simulink model "Sensorverwerking_case1"  (R2018b)
settings: Solver=VariableStepAuto  StartTime=0.0  StopTime=10.0  RelTol=1e-3
undefined symbols (not defined in the file or in its folder): n, sigbuilder_block, Tsc
libraries: dspswit3 x10, simulink x7, powerlib_meascontrol x4, dspsigops x4, peGeneralControl x1
settings Model: Creator=Roberto  LastModifiedBy=Roberto

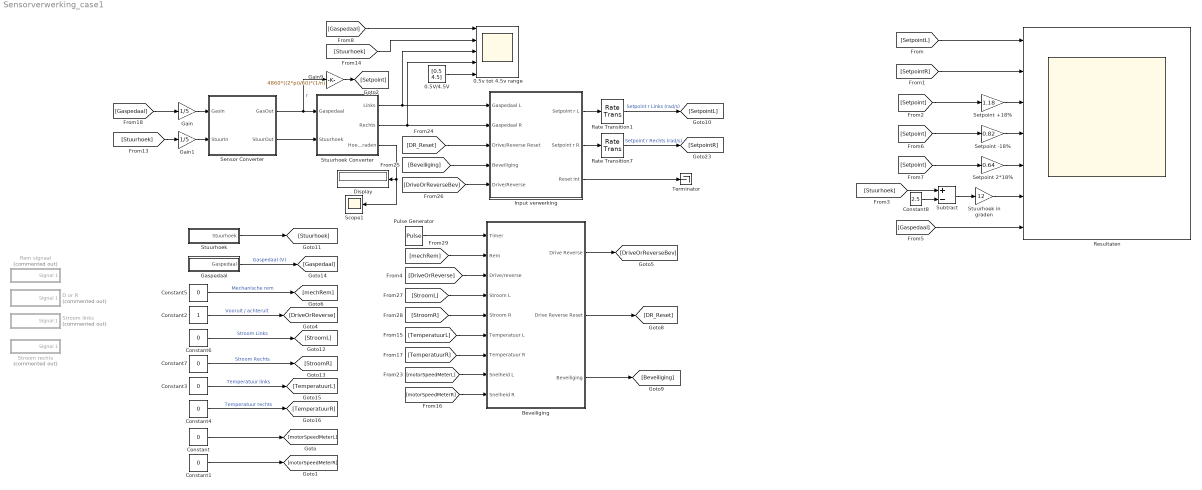
== system Sensorverwerking_case1 ==
  0.5V/4.5V : Constant  Value=[0.5 4.5]
  0.5v tot 4.5v range : Scope  NumInputPorts=5
  Beveiliging : Subsystem
  Constant{,1,3..7} (7 alike) : Constant  Value=0
  Constant2 : Constant
  Constant8 : Constant  Value=2.5
  D or R : Subsystem  Tag=STV Subsys  Commented=on  LoadFcn=sigbuilder_block('load');  StartFcn=sigbuilder_block('start');  StopFcn=sigbuilder_block('stop');  ClipboardFcn=sigbuilder_block('clipboard');  mask(Sigbuilder block){tuvar=[0:10]}
      mask help: Simulink:masks:SigbuilderBlock_MD
      mask init:
      | if ~strcmp(get_param(bdroot(gcbh),'SimulationStatus'),'stopped') tuvar = sigbuilder_block('maskInit'); end
      settings: CopyFcn=sigbuilder_block('copy');  DeleteFcn=sigbuilder_block('delete');  ModelCloseFcn=sigbuilder_block('modelClose');  PreSaveFcn=sigbuilder_block('preSave');  PauseFcn=sigbuilder_block('pause');  ContinueFcn=sigbuilder_block('continue');  NameChangeFcn=sigbuilder_block('namechange');  OpenFcn=sigbuilder_block('open',[437.6 153 550.4 359.25 ]);  CloseFcn=sigbuilder_block('close');
      mask Display: plot(0, 0, 100, 100,[2, 2, 32, 32, 2], [68, 8, 8, 68, 68],[32, 2], [38, 38], [32, 19, 2],[53, 60, 44], [32, 17, 17, 2],[16, 16, 31, 31]);txt = getActiveGroup(gcbh);text(2, 100, txt,'verticalAlignment', 'top');
  Display : Display
  Gain : Gain  Gain=1/5
  Gain1 : Gain  Gain=1/5
  Gain9 : Gain  Gain=4860*((2*pi)/60)*(1/n)
  Gaspedaal : Subsystem  Tag=STV Subsys  LoadFcn=sigbuilder_block('load');  StartFcn=sigbuilder_block('start');  StopFcn=sigbuilder_block('stop');  ClipboardFcn=sigbuilder_block('clipboard');  mask(Sigbuilder block){tuvar=[0:10]}
      mask help: Simulink:masks:SigbuilderBlock_MD
      mask init:
      | if ~strcmp(get_param(bdroot(gcbh),'SimulationStatus'),'stopped') tuvar = sigbuilder_block('maskInit'); end
      settings: CopyFcn=sigbuilder_block('copy');  DeleteFcn=sigbuilder_block('delete');  ModelCloseFcn=sigbuilder_block('modelClose');  PreSaveFcn=sigbuilder_block('preSave');  PauseFcn=sigbuilder_block('pause');  ContinueFcn=sigbuilder_block('continue');  NameChangeFcn=sigbuilder_block('namechange');  OpenFcn=sigbuilder_block('open',[468 234 550.5 278.25 ]);  CloseFcn=sigbuilder_block('close');
      mask Display: plot(0, 0, 100, 100,[2, 2, 32, 32, 2], [68, 8, 8, 68, 68],[32, 2], [38, 38], [32, 19, 2],[53, 60, 44], [32, 17, 17, 2],[16, 16, 31, 31]);txt = getActiveGroup(gcbh);text(2, 100, txt,'verticalAlignment', 'top');
  Input verwerking : Subsystem
  Pulse Generator : DiscretePulseGenerator  SampleTime=1/2000
  Rate Transition1 : RateTransition  OutPortSampleTime=Tsc
  Rate Transition7 : RateTransition  OutPortSampleTime=Tsc
  Rem signaal : Subsystem  Tag=STV Subsys  Commented=on  LoadFcn=sigbuilder_block('load');  StartFcn=sigbuilder_block('start');  StopFcn=sigbuilder_block('stop');  ClipboardFcn=sigbuilder_block('clipboard');  mask(Sigbuilder block){tuvar=[0:10]}
      mask help: Simulink:masks:SigbuilderBlock_MD
      mask init:
      | if ~strcmp(get_param(bdroot(gcbh),'SimulationStatus'),'stopped') tuvar = sigbuilder_block('maskInit'); end
      settings: CopyFcn=sigbuilder_block('copy');  DeleteFcn=sigbuilder_block('delete');  ModelCloseFcn=sigbuilder_block('modelClose');  PreSaveFcn=sigbuilder_block('preSave');  PauseFcn=sigbuilder_block('pause');  ContinueFcn=sigbuilder_block('continue');  NameChangeFcn=sigbuilder_block('namechange');  OpenFcn=sigbuilder_block('open',[437.6 153 550.4 359.25 ]);  CloseFcn=sigbuilder_block('close');
      mask Display: plot(0, 0, 100, 100,[2, 2, 32, 32, 2], [68, 8, 8, 68, 68],[32, 2], [38, 38], [32, 19, 2],[53, 60, 44], [32, 17, 17, 2],[16, 16, 31, 31]);txt = getActiveGroup(gcbh);text(2, 100, txt,'verticalAlignment', 'top');
  Resultaten : Scope  NumInputPorts=7
  Scope1 : Scope
  Sensor Converter : Subsystem
  Setpoint +18% : Gain  Gain=1.18
  Setpoint -18% : Gain  Gain=0.82
  Setpoint 2*18% : Gain  Gain=0.64
  Stroom links : Subsystem  Tag=STV Subsys  Commented=on  LoadFcn=sigbuilder_block('load');  StartFcn=sigbuilder_block('start');  StopFcn=sigbuilder_block('stop');  ClipboardFcn=sigbuilder_block('clipboard');  mask(Sigbuilder block){tuvar=[0:10]}
      mask help: Simulink:masks:SigbuilderBlock_MD
      mask init:
      | if ~strcmp(get_param(bdroot(gcbh),'SimulationStatus'),'stopped') tuvar = sigbuilder_block('maskInit'); end
      settings: CopyFcn=sigbuilder_block('copy');  DeleteFcn=sigbuilder_block('delete');  ModelCloseFcn=sigbuilder_block('modelClose');  PreSaveFcn=sigbuilder_block('preSave');  PauseFcn=sigbuilder_block('pause');  ContinueFcn=sigbuilder_block('continue');  NameChangeFcn=sigbuilder_block('namechange');  OpenFcn=sigbuilder_block('open',[437.6 153 550.4 359.25 ]);  CloseFcn=sigbuilder_block('close');
      mask Display: plot(0, 0, 100, 100,[2, 2, 32, 32, 2], [68, 8, 8, 68, 68],[32, 2], [38, 38], [32, 19, 2],[53, 60, 44], [32, 17, 17, 2],[16, 16, 31, 31]);txt = getActiveGroup(gcbh);text(2, 100, txt,'verticalAlignment', 'top');
  Stroom rechts : Subsystem  Tag=STV Subsys  Commented=on  LoadFcn=sigbuilder_block('load');  StartFcn=sigbuilder_block('start');  StopFcn=sigbuilder_block('stop');  ClipboardFcn=sigbuilder_block('clipboard');  mask(Sigbuilder block){tuvar=[0:10]}
      mask help: Simulink:masks:SigbuilderBlock_MD
      mask init:
      | if ~strcmp(get_param(bdroot(gcbh),'SimulationStatus'),'stopped') tuvar = sigbuilder_block('maskInit'); end
      settings: CopyFcn=sigbuilder_block('copy');  DeleteFcn=sigbuilder_block('delete');  ModelCloseFcn=sigbuilder_block('modelClose');  PreSaveFcn=sigbuilder_block('preSave');  PauseFcn=sigbuilder_block('pause');  ContinueFcn=sigbuilder_block('continue');  NameChangeFcn=sigbuilder_block('namechange');  OpenFcn=sigbuilder_block('open',[437.6 153 550.4 359.25 ]);  CloseFcn=sigbuilder_block('close');
      mask Display: plot(0, 0, 100, 100,[2, 2, 32, 32, 2], [68, 8, 8, 68, 68],[32, 2], [38, 38], [32, 19, 2],[53, 60, 44], [32, 17, 17, 2],[16, 16, 31, 31]);txt = getActiveGroup(gcbh);text(2, 100, txt,'verticalAlignment', 'top');
  Stuurhoek : Subsystem  Tag=STV Subsys  LoadFcn=sigbuilder_block('load');  StartFcn=sigbuilder_block('start');  StopFcn=sigbuilder_block('stop');  ClipboardFcn=sigbuilder_block('clipboard');  mask(Sigbuilder block){tuvar=[0:10]}
      mask help: Simulink:masks:SigbuilderBlock_MD
      mask init:
      | if ~strcmp(get_param(bdroot(gcbh),'SimulationStatus'),'stopped') tuvar = sigbuilder_block('maskInit'); end
      settings: CopyFcn=sigbuilder_block('copy');  DeleteFcn=sigbuilder_block('delete');  ModelCloseFcn=sigbuilder_block('modelClose');  PreSaveFcn=sigbuilder_block('preSave');  PauseFcn=sigbuilder_block('pause');  ContinueFcn=sigbuilder_block('continue');  NameChangeFcn=sigbuilder_block('namechange');  OpenFcn=sigbuilder_block('open',[1567.5 274.5 552.75 320.25 ]);  CloseFcn=sigbuilder_block('close');
      mask Display: plot(0, 0, 100, 100,[2, 2, 32, 32, 2], [68, 8, 8, 68, 68],[32, 2], [38, 38], [32, 19, 2],[53, 60, 44], [32, 17, 17, 2],[16, 16, 31, 31]);txt = getActiveGroup(gcbh);text(2, 100, txt,'verticalAlignment', 'top');
  Stuurhoek Converter : Subsystem
  Stuurhoek in graden : Gain  Gain=12
  Subtract : Sum  Inputs=+-
  Terminator : Terminator
  wires:
  Input verwerking/2(Setpoint r R) -> Rate Transition7/1
  Stuurhoek Converter/1(Links) -> Input verwerking/1(Gaspedaal L), 0.5v tot 4.5v range/3
  Rate Transition7/1 -> [SetpointR]  "Setpoint r Rechts (rad/s)"
  Stuurhoek Converter/2(Rechts) -> 0.5v tot 4.5v range/4, Input verwerking/2(Gaspedaal R)
  [Gaspedaal] -> Gain/1
  [Beveiliging] -> Input verwerking/4(Beveiliging)
  Input verwerking/1(Setpoint r L) -> Rate Transition1/1
  [DriveOrReverseBev] -> Input verwerking/5(Drive/Reverse)
  Input verwerking/3(Reset Int) -> Terminator/1
  [Stuurhoek] -> Gain1/1
  [DR_Reset] -> Input verwerking/3(Drive/Reverse Reset)
  Rate Transition1/1 -> [SetpointL]  "Setpoint r Links (rad/s)"
  Beveiliging/2(Drive Reverse Reset) -> [DR_Reset]
  Pulse Generator/1 -> Beveiliging/1(Timer)
  [TemperatuurR] -> Beveiliging/7(Temperatuur R)
  [StroomR] -> Beveiliging/5(Stroom R)
  [mechRem] -> Beveiliging/2(Rem)
  [motorSpeedMeterL] -> Beveiliging/8(Snelheid L)
  Beveiliging/1("Drive Reverse ") -> [DriveOrReverseBev]
  [TemperatuurL] -> Beveiliging/6(Temperatuur L)
  [motorSpeedMeterR] -> Beveiliging/9(Snelheid R)
  [DriveOrReverse] -> Beveiliging/3(Drive/reverse)
  [StroomL] -> Beveiliging/4(Stroom L)
  Beveiliging/3(Beveiliging) -> [Beveiliging]
  Constant3/1 -> [TemperatuurL]  "Temperatuur links"
  Constant5/1 -> [mechRem]  "Mechanische rem"
  Constant4/1 -> [TemperatuurR]  "Temperatuur rechts"
  Constant2/1 -> [DriveOrReverse]  "Vooruit / achteruit"
  Constant7/1 -> [StroomR]  "Stroom Rechts"
  Constant6/1 -> [StroomL]  "Stroom Links"
  Sensor Converter/2(StuurOut) -> Stuurhoek Converter/2(Stuurhoek)
  [Stuurhoek] -> 0.5v tot 4.5v range/2
  Gaspedaal/1(Gaspedaal) -> [Gaspedaal]  "Gaspedaal (V)"
  Gain/1 -> Sensor Converter/1(GasIn)
  0.5V/4.5V/1 -> 0.5v tot 4.5v range/5
  Gain1/1 -> Sensor Converter/2(StuurIn)
  Stuurhoek/1(Stuurhoek) -> [Stuurhoek]
  Stuurhoek Converter/3(Hoek in graden) -> Scope1/1, Display/1
  [Gaspedaal] -> 0.5v tot 4.5v range/1
  [Gaspedaal] -> Resultaten/7
  Constant/1 -> [motorSpeedMeterL]
  Constant1/1 -> [motorSpeedMeterR]
  [Stuurhoek] -> Subtract/1
  Stuurhoek in graden/1 -> Resultaten/6
  Subtract/1 -> Stuurhoek in graden/1
  Constant8/1 -> Subtract/2
  [SetpointL] -> Resultaten/1
  Setpoint -18%/1 -> Resultaten/4
  [Setpoint] -> Setpoint +18%/1
  Setpoint +18%/1 -> Resultaten/3
  [SetpointR] -> Resultaten/2
  [Setpoint] -> Setpoint -18%/1
  [Setpoint] -> Setpoint 2*18%/1
  Setpoint 2*18%/1 -> Resultaten/5
  Gain9/1 -> [Setpoint]
  Sensor Converter/1(GasOut) -> Gain9/1, Stuurhoek Converter/1("Gaspedaal ")  "r"

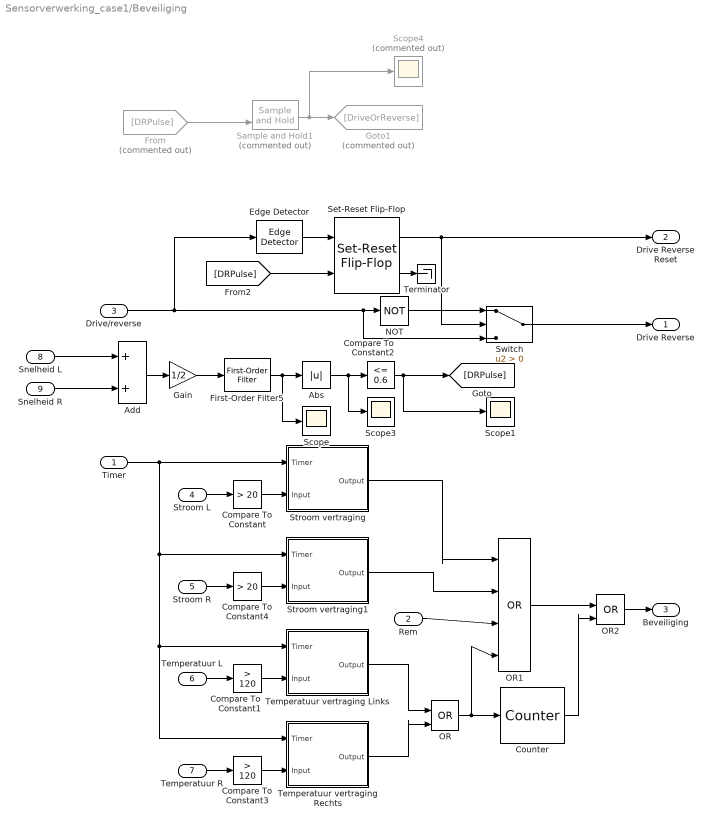
== system Sensorverwerking_case1/Beveiliging ==
  Timer : Inport
  Rem : Inport  Port=2
  Drive/reverse : Inport  Port=3
  Stroom L : Inport  Port=4
  Stroom R : Inport  Port=5
  Temperatuur L : Inport  Port=6
  Temperatuur R : Inport  Port=7
  Snelheid L : Inport  Port=8
  Snelheid R : Inport  Port=9
  Abs : Abs
  Add : Sum
  Compare To Constant : simulink/Logic and Bit Operations/Compare To Constant  relop=>  const=20  OutDataTypeStr=boolean
  Compare To Constant1 : simulink/Logic and Bit Operations/Compare To Constant  relop=>  const=120  OutDataTypeStr=boolean
  Compare To Constant2 : simulink/Logic and Bit Operations/Compare To Constant  relop=<=  const=0.6  OutDataTypeStr=boolean
  Compare To Constant3 : simulink/Logic and Bit Operations/Compare To Constant  relop=>  const=120  OutDataTypeStr=boolean
  Compare To Constant4 : simulink/Logic and Bit Operations/Compare To Constant  relop=>  const=20  OutDataTypeStr=boolean
  Counter : dspswit3/Counter  Direction=Up  CountEvent=Rising edge  CounterSize=32 bits  MaxCount=255  InitialCount=0  Output=Hit  HitValue=3  ResetInput=off  SamplesPerFrame=1  Ts=1  CntDtype=double  HitDtype=Logical
  Edge Detector : powerlib_meascontrol/Logic/Edge Detector  model=Either  ic=0  Ts=-1
      settings: SourceProductName=Simscape Power Systems  SourceProductBaseCode=PS
  First-Order Filter5 : powerlib_meascontrol/Filters/First-Order Filter  FilterType=Lowpass  Tc=10e-3  Ts=Tsc  Initialize=on  Vac_Init=[0, 0, 50]  Vdc_Init=0  PlotResponse=off  FreqRange="[0,  200,  1]"
      settings: SourceProductName=Simscape Power Systems
  From : From  Commented=on  GotoTag=DRPulse
  Gain : Gain  Gain=1/2
  Goto1 : Goto  Commented=on  GotoTag=DriveOrReverse
  NOT : Logic  Operator=NOT  IconShape=distinctive  AllPortsSameDT=off  OutDataTypeStr=boolean
  OR : Logic  Operator=OR  IconShape=distinctive  AllPortsSameDT=off  OutDataTypeStr=boolean
  OR1 : Logic  Operator=OR  Inputs=4  IconShape=distinctive  AllPortsSameDT=off  OutDataTypeStr=boolean
  OR2 : Logic  Operator=OR  IconShape=distinctive  AllPortsSameDT=off  OutDataTypeStr=boolean
  Sample and Hold1 : powerlib_meascontrol/Additional Components/Sample and Hold  Commented=on  ic=0  Ts=0
      settings: SourceProductName=Simscape Power Systems  SourceProductBaseCode=PS
  Scope : Scope
  Scope1 : Scope
  Scope3 : Scope
  Scope4 : Scope  Commented=on
  Set-Reset Flip-Flop : peGeneralControl/Set-Reset Flip-Flop  LabelModeActiveChoice=Discrete  UndefState=Set  Q0=0  Ts=-1
  Stroom vertraging : Subsystem
  Stroom vertraging1 : Subsystem
  Switch : Switch  Criteria=u2 > Threshold
  Temperatuur vertraging Links : Subsystem
  Temperatuur vertraging Rechts : Subsystem
  Terminator : Terminator
  "Drive Reverse " : Outport
  Drive Reverse Reset : Outport  Port=2
  Beveiliging : Outport  Port=3
  wires:
  Compare To Constant/1 -> Stroom vertraging/2(Input)
  Stroom L/1 -> Compare To Constant/1
  Compare To Constant1/1 -> Temperatuur vertraging Links/2(Input)
  Temperatuur L/1 -> Compare To Constant1/1
  Edge Detector/1 -> Set-Reset Flip-Flop/1
  Set-Reset Flip-Flop/1 -> Switch/2, Drive Reverse Reset/1
  Sample and Hold1/1 -> Scope4/1, Goto1/1
  Abs/1 -> Scope3/1, Compare To Constant2/1
  Compare To Constant2/1 -> [DRPulse], Scope1/1
  [DRPulse] -> Set-Reset Flip-Flop/2
  Drive/reverse/1 -> Edge Detector/1, Switch/3, NOT/1
  From/1 -> Sample and Hold1/2
  Snelheid L/1 -> Add/1
  Snelheid R/1 -> Add/2
  Add/1 -> Gain/1
  Gain/1 -> First-Order Filter5/1
  Compare To Constant3/1 -> Temperatuur vertraging Rechts/2(Input)
  Timer/1 -> Stroom vertraging1/1(Timer), Temperatuur vertraging Rechts/1(Timer), Temperatuur vertraging Links/1(Timer), Stroom vertraging/1(Timer)
  Compare To Constant4/1 -> Stroom vertraging1/2(Input)
  Stroom R/1 -> Compare To Constant4/1
  Rem/1 -> OR1/3
  Stroom vertraging/1(Output) -> OR1/1
  Stroom vertraging1/1(Output) -> OR1/2
  Switch/1 -> "Drive Reverse "/1
  NOT/1 -> Switch/1
  OR/1 -> OR1/4, Counter/1
  Temperatuur vertraging Links/1(Output) -> OR/1
  Temperatuur vertraging Rechts/1(Output) -> OR/2
  OR2/1 -> Beveiliging/1
  Counter/1 -> OR2/2
  OR1/1 -> OR2/1
  Temperatuur R/1 -> Compare To Constant3/1
  Set-Reset Flip-Flop/2 -> Terminator/1
  First-Order Filter5/1 -> Scope/1, Abs/1

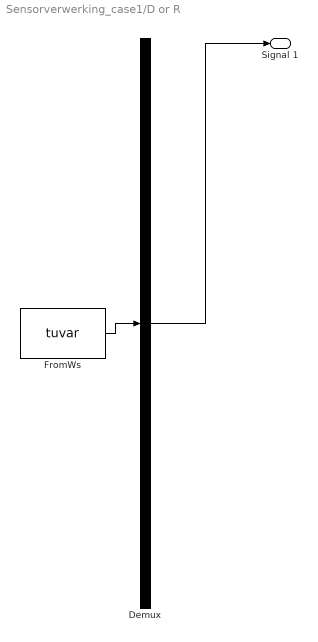
== system Sensorverwerking_case1/D or R ==
  Demux : Demux  Tag=STV Demux  Outputs=1
  FromWs : FromWorkspace  Tag=STV FromWs  VariableName=tuvar  SampleTime=0
      SigBuilderData=|
      | common.afterFinalStr = 'Extrapolate'
      | common.sampleTime = 0
      | dataSet.timeRange = [0 10]
      | dataSet.name = 'Group 1'
      | sbobj.Groups.Name = 'Group 1'
      | sbobj.Groups.Signals.Name = 'Signal 1'
      | sbobj.Groups.Signals.XData = [0 2 2 4 4 6.5 6.5 9.6 9.6 10]
      | sbobj.Groups.Signals.YData = [0 0 1 1 0 0 1 1 0 0]
  Signal 1 : Outport  Tag=STV Outport
  wires:
  Demux/1 -> Signal 1/1
  FromWs/1 -> Demux/1

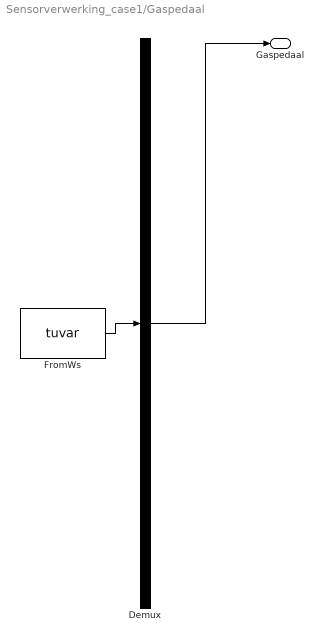
== system Sensorverwerking_case1/Gaspedaal ==
  Demux : Demux  Tag=STV Demux  Outputs=1
  FromWs : FromWorkspace  Tag=STV FromWs  VariableName=tuvar  SampleTime=0
      SigBuilderData=|
      | common.afterFinalStr = 'Extrapolate'
      | common.sampleTime = 0
      | dataSet.timeRange = [0 10]
      | dataSet.name = 'Group 1'
      | sbobj.Groups.Name = 'Group 1'
      | sbobj.Groups.Signals.Name = 'Gaspedaal'
      | sbobj.Groups.Signals.XData = [0 2 4 4 7 7 10]
      | sbobj.Groups.Signals.YData = [0 5 0 2 2 5 5]
  Gaspedaal : Outport  Tag=STV Outport
  wires:
  Demux/1 -> Gaspedaal/1
  FromWs/1 -> Demux/1

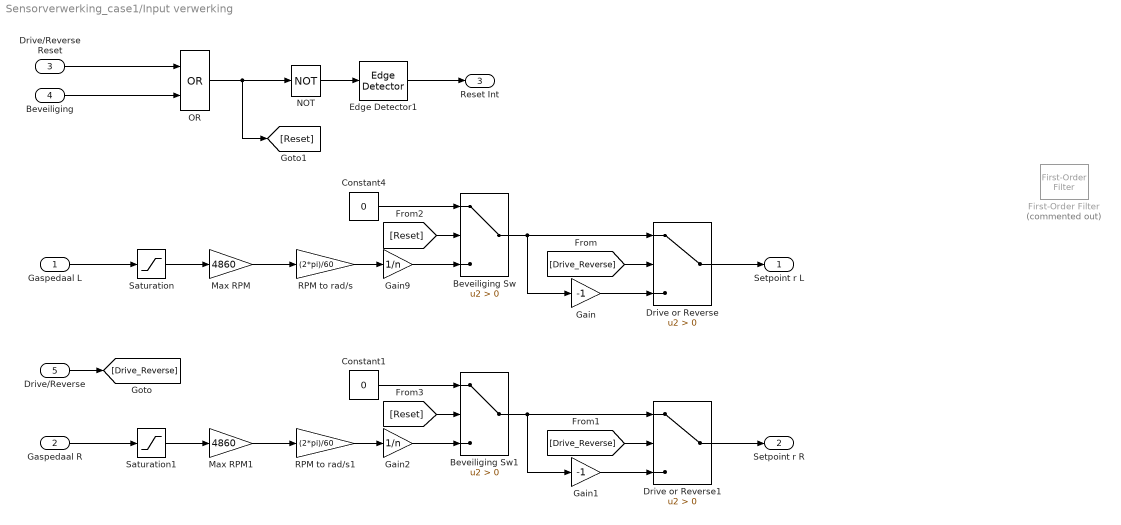
== system Sensorverwerking_case1/Input verwerking ==
  Gaspedaal L : Inport
  Gaspedaal R : Inport  Port=2
  Drive/Reverse Reset : Inport  Port=3
  Beveiliging : Inport  Port=4
  Drive/Reverse : Inport  Port=5
  Beveiliging Sw : Switch  Criteria=u2 > Threshold
  Beveiliging Sw1 : Switch  Criteria=u2 > Threshold
  Constant1 : Constant  Value=0
  Constant4 : Constant  Value=0
  Drive or Reverse : Switch  Criteria=u2 > Threshold
  Drive or Reverse1 : Switch  Criteria=u2 > Threshold
  Edge Detector1 : dspswit3/Edge Detector  InputProcessing=Columns as channels (frame based)
      settings: SourceProductName=DSP System Toolbox  SourceProductBaseCode=DS
  First-Order Filter : powerlib_meascontrol/Filters/First-Order Filter  Commented=on  FilterType=Lowpass  Tc=10e-2  Ts=0  Initialize=on  Vac_Init=[0, 0, 60]  Vdc_Init=0  PlotResponse=off  FreqRange="[0,  200,  1]"
      settings: SourceProductName=Simscape Power Systems
  Gain : Gain  Gain=-1
  Gain1 : Gain  Gain=-1
  Gain2 : Gain  Gain=1/n
  Gain9 : Gain  Gain=1/n
  Max RPM : Gain  Gain=4860
  Max RPM1 : Gain  Gain=4860
  NOT : Logic  Operator=NOT  IconShape=distinctive  AllPortsSameDT=off  OutDataTypeStr=boolean
  OR : Logic  Operator=OR  IconShape=distinctive  AllPortsSameDT=off  OutDataTypeStr=boolean
  RPM to rad/s : Gain  Gain=(2*pi)/60
  RPM to rad/s1 : Gain  Gain=(2*pi)/60
  Saturation : Saturate  UpperLimit=inf  LowerLimit=0
  Saturation1 : Saturate  UpperLimit=inf  LowerLimit=0
  Setpoint r L : Outport
  Setpoint r R : Outport  Port=2
  Reset Int : Outport  Port=3
  wires:
  Constant4/1 -> Beveiliging Sw/1
  Max RPM/1 -> RPM to rad/s/1
  Saturation/1 -> Max RPM/1
  RPM to rad/s/1 -> Gain9/1
  Gaspedaal L/1 -> Saturation/1
  OR/1 -> [Reset], NOT/1
  Gain9/1 -> Beveiliging Sw/3
  Beveiliging Sw/1 -> Gain/1, Drive or Reverse/1
  Gain/1 -> Drive or Reverse/3
  [Drive_Reverse] -> Drive or Reverse/2
  Drive or Reverse/1 -> Setpoint r L/1
  Edge Detector1/1 -> Reset Int/1
  NOT/1 -> Edge Detector1/1
  Beveiliging/1 -> OR/2
  Drive/Reverse Reset/1 -> OR/1
  Max RPM1/1 -> RPM to rad/s1/1
  Saturation1/1 -> Max RPM1/1
  RPM to rad/s1/1 -> Gain2/1
  Drive or Reverse1/1 -> Setpoint r R/1
  Gaspedaal R/1 -> Saturation1/1
  Gain1/1 -> Drive or Reverse1/3
  Beveiliging Sw1/1 -> Gain1/1, Drive or Reverse1/1
  Constant1/1 -> Beveiliging Sw1/1
  [Drive_Reverse] -> Drive or Reverse1/2
  Gain2/1 -> Beveiliging Sw1/3
  Drive/Reverse/1 -> [Drive_Reverse]
  [Reset] -> Beveiliging Sw/2
  [Reset] -> Beveiliging Sw1/2

== system Sensorverwerking_case1/Rem signaal ==
  Demux : Demux  Tag=STV Demux  Outputs=1
  FromWs : FromWorkspace  Tag=STV FromWs  VariableName=tuvar  SampleTime=0
      SigBuilderData=|
      | common.afterFinalStr = 'Extrapolate'
      | common.sampleTime = 0
      | dataSet.timeRange = [0 10]
      | dataSet.name = 'Group 1'
      | sbobj.Groups.Name = 'Group 1'
      | sbobj.Groups.Signals.Name = 'Signal 1'
      | sbobj.Groups.Signals.XData = [0 6 6 7 7 9 9 9.6 9.6 10]
      | sbobj.Groups.Signals.YData = [0 0 1 1 0 0 1 1 0 0]
  Signal 1 : Outport  Tag=STV Outport
  wires:
  Demux/1 -> Signal 1/1
  FromWs/1 -> Demux/1

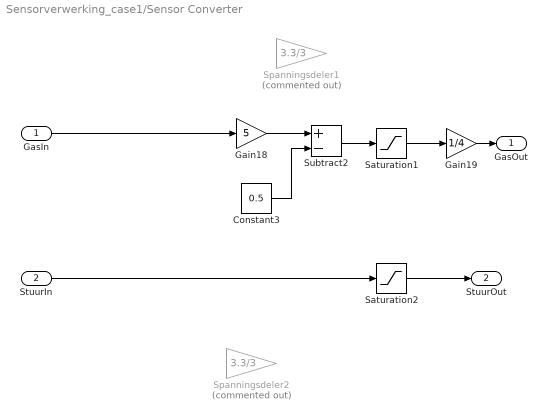
== system Sensorverwerking_case1/Sensor Converter ==
  GasIn : Inport
  StuurIn : Inport  Port=2
  Constant3 : Constant  Value=0.5
  Gain18 : Gain  Gain=5
  Gain19 : Gain  Gain=1/4
  Saturation1 : Saturate  UpperLimit=4  LowerLimit=0
  Saturation2 : Saturate  UpperLimit=1  LowerLimit=0
  Spanningsdeler1 : Gain  Commented=on  Gain=3.3/3
  Spanningsdeler2 : Gain  Commented=on  Gain=3.3/3
  Subtract2 : Sum  Inputs=+-
  GasOut : Outport
  StuurOut : Outport  Port=2
  wires:
  Constant3/1 -> Subtract2/2
  Saturation1/1 -> Gain19/1
  GasIn/1 -> Gain18/1
  Gain18/1 -> Subtract2/1
  Gain19/1 -> GasOut/1
  Subtract2/1 -> Saturation1/1
  Saturation2/1 -> StuurOut/1
  StuurIn/1 -> Saturation2/1

== system Sensorverwerking_case1/Stroom links ==
  Demux : Demux  Tag=STV Demux  Outputs=1
  FromWs : FromWorkspace  Tag=STV FromWs  VariableName=tuvar  SampleTime=0
      SigBuilderData=|
      | common.afterFinalStr = 'Extrapolate'
      | common.sampleTime = 0
      | dataSet.timeRange = [0 10]
      | dataSet.name = 'Group 1'
      | sbobj.Groups.Name = 'Group 1'
      | sbobj.Groups.Signals.Name = 'Signal 1'
      | sbobj.Groups.Signals.XData = [0 1 1.5 2 7 10]
      | sbobj.Groups.Signals.YData = [0 0 30 0 0 0]
  Signal 1 : Outport  Tag=STV Outport
  wires:
  Demux/1 -> Signal 1/1
  FromWs/1 -> Demux/1

== system Sensorverwerking_case1/Stroom rechts ==
  Demux : Demux  Tag=STV Demux  Outputs=1
  FromWs : FromWorkspace  Tag=STV FromWs  VariableName=tuvar  SampleTime=0
      SigBuilderData=|
      | common.afterFinalStr = 'Extrapolate'
      | common.sampleTime = 0
      | dataSet.timeRange = [0 10]
      | dataSet.name = 'Group 1'
      | sbobj.Groups.Name = 'Group 1'
      | sbobj.Groups.Signals.Name = 'Signal 1'
      | sbobj.Groups.Signals.XData = [0 1 1.5 2 7 10]
      | sbobj.Groups.Signals.YData = [0 0 30 0 0 0]
  Signal 1 : Outport  Tag=STV Outport
  wires:
  Demux/1 -> Signal 1/1
  FromWs/1 -> Demux/1

== system Sensorverwerking_case1/Stuurhoek ==
  Demux : Demux  Tag=STV Demux  Outputs=1
  FromWs : FromWorkspace  Tag=STV FromWs  VariableName=tuvar  SampleTime=0
      SigBuilderData=|
      | common.afterFinalStr = 'Extrapolate'
      | common.sampleTime = 0
      | dataSet.timeRange = [0 10]
      | dataSet.name = 'Group 1'
      | sbobj.Groups.Name = 'Group 1'
      | sbobj.Groups.Signals.Name = 'Stuurhoek'
      | sbobj.Groups.Signals.XData = [0 4 5 6 7 8 9 10]
      | sbobj.Groups.Signals.YData = [2.5 2.5 5 0 2.5 5 0 2.5]
  Stuurhoek : Outport  Tag=STV Outport
  wires:
  Demux/1 -> Stuurhoek/1
  FromWs/1 -> Demux/1

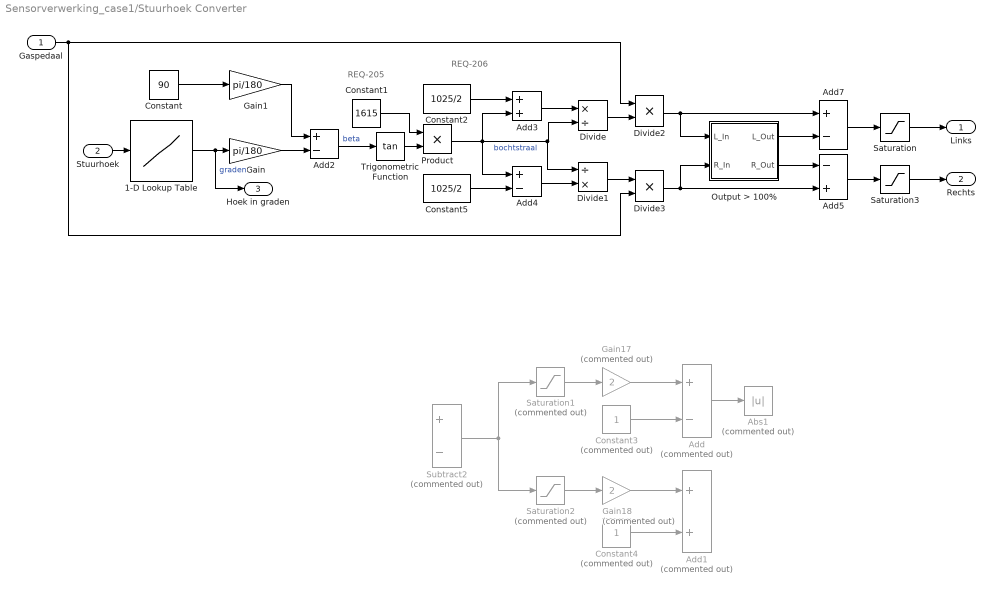
== system Sensorverwerking_case1/Stuurhoek Converter ==
  note: REQ-205
  note: REQ-206
  "Gaspedaal " : Inport
  Stuurhoek : Inport  Port=2
  1-D Lookup Table : Lookup_n-D  NumberOfTableDimensions=1  BreakpointsForDimension1=[0 0.5 1]  Table=[-30 0 30]  InternalRulePriority=Speed  RndMeth=Simplest  InputSameDT=on
  Abs1 : Abs  Commented=on
  Add : Sum  Commented=on  Inputs=+-
  Add1 : Sum  Commented=on
  Add2 : Sum  Inputs=+-
  Add3 : Sum
  Add4 : Sum  Inputs=+-
  Add5 : Sum  Inputs=-+
  Add7 : Sum  Inputs=+-
  Constant : Constant  Value=90
  Constant1 : Constant  Value=1615
  Constant2 : Constant  Value=1025/2
  Constant3 : Constant  Commented=on
  Constant4 : Constant  Commented=on
  Constant5 : Constant  Value=1025/2
  Divide : Product  Inputs=*/
  Divide1 : Product  Inputs=/*
  Divide2 : Product  Inputs=**
  Divide3 : Product  Inputs=**
  Gain : Gain  Gain=pi/180
  Gain1 : Gain  Gain=pi/180
  Gain17 : Gain  Commented=on  Gain=2
  Gain18 : Gain  Commented=on  Gain=2
  Output > 100% : Subsystem
  Product : Product
  Saturation : Saturate  UpperLimit=1  LowerLimit=0
  Saturation1 : Saturate  Commented=on  LowerLimit=0
  Saturation2 : Saturate  Commented=on  UpperLimit=0
  Saturation3 : Saturate  UpperLimit=1  LowerLimit=0
  Subtract2 : Sum  Commented=on  Inputs=+-
  Trigonometric Function : Trigonometry  Operator=tan
  Links : Outport
  Rechts : Outport  Port=2
  Hoek in graden : Outport  Port=3
  wires:
  Saturation1/1 -> Gain17/1
  Subtract2/1 -> Saturation2/1, Saturation1/1
  Gain18/1 -> Add1/1
  Add/1 -> Abs1/1
  Saturation2/1 -> Gain18/1
  Gain17/1 -> Add/1
  Constant4/1 -> Add1/2
  Constant3/1 -> Add/2
  1-D Lookup Table/1 -> Hoek in graden/1, Gain/1  "graden"
  Constant/1 -> Gain1/1
  Add2/1 -> Trigonometric Function/1  "beta"
  Constant1/1 -> Product/1
  Trigonometric Function/1 -> Product/2
  Product/1 -> Divide1/1, Divide/2, Add4/1, Add3/2  "bochtstraal"
  Constant2/1 -> Add3/1
  Add3/1 -> Divide/1
  Constant5/1 -> Add4/2
  Add4/1 -> Divide1/2
  Divide1/1 -> Divide3/1
  Divide/1 -> Divide2/2
  "Gaspedaal "/1 -> Divide2/1, Divide3/2
  Divide2/1 -> Add7/1, Output > 100%/1(L_In)
  Divide3/1 -> Output > 100%/2(R_In), Add5/2
  Stuurhoek/1 -> 1-D Lookup Table/1
  Gain/1 -> Add2/2
  Gain1/1 -> Add2/1
  Add7/1 -> Saturation/1
  Add5/1 -> Saturation3/1
  Output > 100%/1(L_Out) -> Add7/2
  Output > 100%/2(R_Out) -> Add5/1
  Saturation/1 -> Links/1
  Saturation3/1 -> Rechts/1

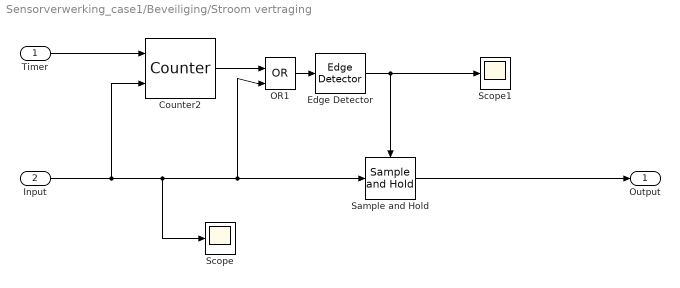
== system Sensorverwerking_case1/Beveiliging/Stroom vertraging ==
  Timer : Inport
  Input : Inport  Port=2
  Counter2 : dspswit3/Counter  Direction=Up  CountEvent=Rising edge  CounterSize=User defined  MaxCount=300  InitialCount=0  Output=Hit  HitValue=300  ResetInput=on  SamplesPerFrame=1  Ts=1  CntDtype=double  HitDtype=Logical
  Edge Detector : dspswit3/Edge Detector  InputProcessing=Columns as channels (frame based)
      settings: SourceProductName=DSP System Toolbox  SourceProductBaseCode=DS
  OR1 : Logic  Operator=OR  IconShape=distinctive  AllPortsSameDT=off  OutDataTypeStr=boolean
  Sample and Hold : dspsigops/Sample and Hold  trig=Rising edge  initCond=0  latchinput=off
  Scope : Scope
  Scope1 : Scope
  Output : Outport
  wires:
  Timer/1 -> Counter2/1
  Sample and Hold/1 -> Output/1
  OR1/1 -> Edge Detector/1
  Input/1 -> Counter2/2, Scope/1, OR1/2, Sample and Hold/1
  Edge Detector/1 -> Scope1/1, Sample and Hold/Trigger
  Counter2/1 -> OR1/1

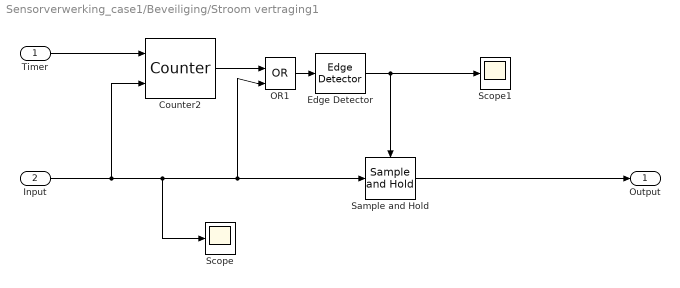
== system Sensorverwerking_case1/Beveiliging/Stroom vertraging1 ==
  Timer : Inport
  Input : Inport  Port=2
  Counter2 : dspswit3/Counter  Direction=Up  CountEvent=Rising edge  CounterSize=User defined  MaxCount=300  InitialCount=0  Output=Hit  HitValue=300  ResetInput=on  SamplesPerFrame=1  Ts=1  CntDtype=double  HitDtype=Logical
  Edge Detector : dspswit3/Edge Detector  InputProcessing=Columns as channels (frame based)
      settings: SourceProductName=DSP System Toolbox  SourceProductBaseCode=DS
  OR1 : Logic  Operator=OR  IconShape=distinctive  AllPortsSameDT=off  OutDataTypeStr=boolean
  Sample and Hold : dspsigops/Sample and Hold  trig=Rising edge  initCond=0  latchinput=off
  Scope : Scope
  Scope1 : Scope
  Output : Outport
  wires:
  Timer/1 -> Counter2/1
  Sample and Hold/1 -> Output/1
  OR1/1 -> Edge Detector/1
  Input/1 -> Counter2/2, Scope/1, OR1/2, Sample and Hold/1
  Edge Detector/1 -> Scope1/1, Sample and Hold/Trigger
  Counter2/1 -> OR1/1

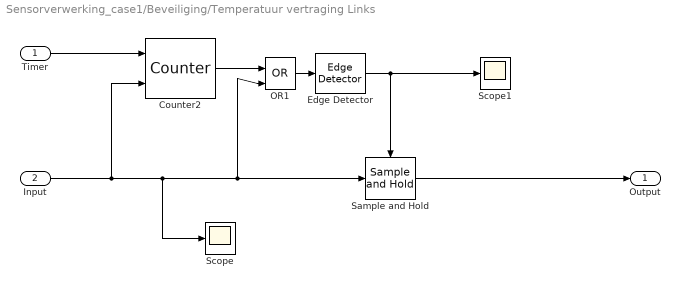
== system Sensorverwerking_case1/Beveiliging/Temperatuur vertraging Links ==
  Timer : Inport
  Input : Inport  Port=2
  Counter2 : dspswit3/Counter  Direction=Up  CountEvent=Rising edge  CounterSize=User defined  MaxCount=30000  InitialCount=0  Output=Hit  HitValue=30000  ResetInput=on  SamplesPerFrame=1  Ts=1  CntDtype=double  HitDtype=Logical
  Edge Detector : dspswit3/Edge Detector  InputProcessing=Columns as channels (frame based)
      settings: SourceProductName=DSP System Toolbox  SourceProductBaseCode=DS
  OR1 : Logic  Operator=OR  IconShape=distinctive  AllPortsSameDT=off  OutDataTypeStr=boolean
  Sample and Hold : dspsigops/Sample and Hold  trig=Rising edge  initCond=0  latchinput=off
  Scope : Scope
  Scope1 : Scope
  Output : Outport
  wires:
  Timer/1 -> Counter2/1
  Sample and Hold/1 -> Output/1
  OR1/1 -> Edge Detector/1
  Input/1 -> Counter2/2, Scope/1, OR1/2, Sample and Hold/1
  Edge Detector/1 -> Scope1/1, Sample and Hold/Trigger
  Counter2/1 -> OR1/1

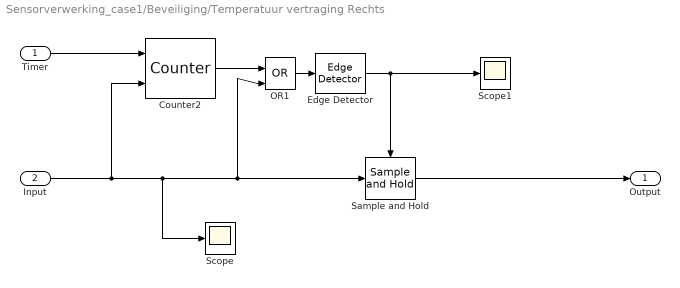
== system Sensorverwerking_case1/Beveiliging/Temperatuur vertraging Rechts ==
  Timer : Inport
  Input : Inport  Port=2
  Counter2 : dspswit3/Counter  Direction=Up  CountEvent=Rising edge  CounterSize=User defined  MaxCount=30000  InitialCount=0  Output=Hit  HitValue=30000  ResetInput=on  SamplesPerFrame=1  Ts=1  CntDtype=double  HitDtype=Logical
  Edge Detector : dspswit3/Edge Detector  InputProcessing=Columns as channels (frame based)
      settings: SourceProductName=DSP System Toolbox  SourceProductBaseCode=DS
  OR1 : Logic  Operator=OR  IconShape=distinctive  AllPortsSameDT=off  OutDataTypeStr=boolean
  Sample and Hold : dspsigops/Sample and Hold  trig=Rising edge  initCond=0  latchinput=off
  Scope : Scope
  Scope1 : Scope
  Output : Outport
  wires:
  Timer/1 -> Counter2/1
  Sample and Hold/1 -> Output/1
  OR1/1 -> Edge Detector/1
  Input/1 -> Counter2/2, Scope/1, OR1/2, Sample and Hold/1
  Edge Detector/1 -> Scope1/1, Sample and Hold/Trigger
  Counter2/1 -> OR1/1

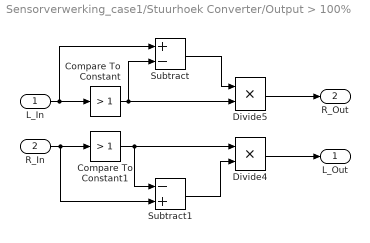
== system Sensorverwerking_case1/Stuurhoek Converter/Output > 100% ==
  L_In : Inport
  R_In : Inport  Port=2
  Compare To Constant : simulink/Logic and Bit Operations/Compare To Constant  relop=>  const=1  OutDataTypeStr=boolean
  Compare To Constant1 : simulink/Logic and Bit Operations/Compare To Constant  relop=>  const=1  OutDataTypeStr=boolean
  Divide4 : Product  Inputs=**
  Divide5 : Product  Inputs=**
  Subtract : Sum  Inputs=+-
  Subtract1 : Sum  Inputs=-+
  L_Out : Outport
  R_Out : Outport  Port=2
  wires:
  Compare To Constant1/1 -> Subtract1/1, Divide4/1
  Compare To Constant/1 -> Subtract/2, Divide5/2
  Subtract1/1 -> Divide4/2
  Subtract/1 -> Divide5/1
  L_In/1 -> Subtract/1, Compare To Constant/1
  Divide5/1 -> R_Out/1
  R_In/1 -> Subtract1/2, Compare To Constant1/1
  Divide4/1 -> L_Out/1
